simulink model "Caso4CicloLimite"  (R2015a)
settings: Solver=ode45  StartTime=0.0  StopTime=10.0  RelTol=1e-3
settings Model: Creator=user  LastModifiedBy=user

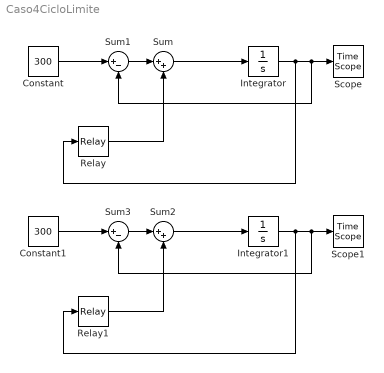
== system Caso4CicloLimite ==
  Constant : Constant  Value=300
  Constant1 : Constant  Value=300
  Integrator : Integrator  InitialCondition=250
  Integrator1 : Integrator  InitialCondition=320
  Relay : Relay  OnSwitchValue=290  OffSwitchValue=287  OnOutputValue=-200
  Relay1 : Relay  OnSwitchValue=290  OffSwitchValue=287  OnOutputValue=-200
  Scope : TimeScope
  Scope1 : TimeScope
  Sum : Sum  Inputs=|++
  Sum1 : Sum  Inputs=|+-
  Sum2 : Sum  Inputs=|++
  Sum3 : Sum  Inputs=|+-
  wires:
  Integrator/1 -> Sum1/2, Scope/1, Relay/1
  Sum/1 -> Integrator/1
  Relay/1 -> Sum/2
  Sum1/1 -> Sum/1
  Constant/1 -> Sum1/1
  Integrator1/1 -> Sum3/2, Scope1/1, Relay1/1
  Sum2/1 -> Integrator1/1
  Relay1/1 -> Sum2/2
  Sum3/1 -> Sum2/1
  Constant1/1 -> Sum3/1
